simulink library "CTRL_SPECCTRL_COND"  (R2024b)
settings: Solver=VariableStepAuto  StartTime=0.0  StopTime=10.0  RelTol=1e-3
settings Model: Creator=blatak  LastModifiedBy=blatak

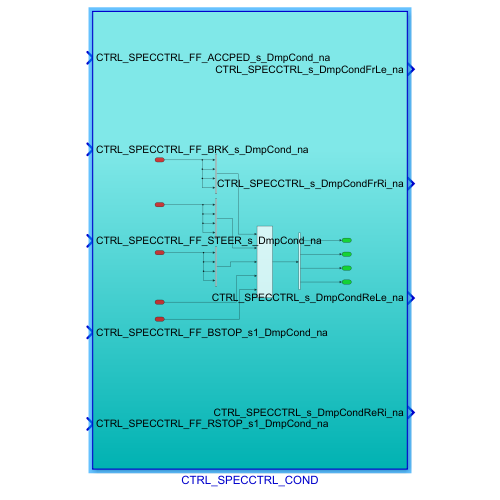
[thumbnail: Simulink's stored preview of the top-level diagram]
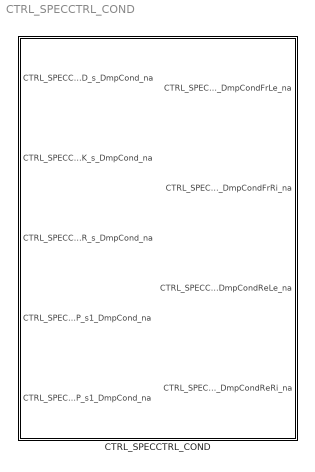
== system CTRL_SPECCTRL_COND ==
  CTRL_SPECCTRL_COND : Subsystem

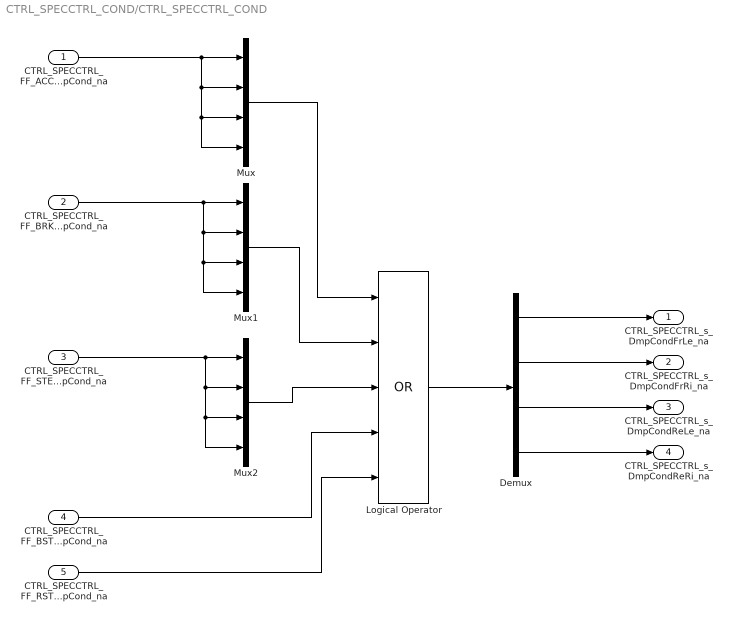
== system CTRL_SPECCTRL_COND/CTRL_SPECCTRL_COND ==
  CTRL_SPECCTRL_FF_ACCPED_s_DmpCond_na : Inport
  CTRL_SPECCTRL_FF_BRK_s_DmpCond_na : Inport  Port=2
  CTRL_SPECCTRL_FF_STEER_s_DmpCond_na : Inport  Port=3
  CTRL_SPECCTRL_FF_BSTOP_s1_DmpCond_na : Inport  Port=4
  CTRL_SPECCTRL_FF_RSTOP_s1_DmpCond_na : Inport  Port=5
  Demux : Demux
  Logical Operator : Logic  Operator=OR  Inputs=5  AllPortsSameDT=off  OutDataTypeStr=boolean
  Mux : Mux
  Mux1 : Mux
  Mux2 : Mux
  CTRL_SPECCTRL_s_DmpCondFrLe_na : Outport
  CTRL_SPECCTRL_s_DmpCondFrRi_na : Outport  Port=2
  CTRL_SPECCTRL_s_DmpCondReLe_na : Outport  Port=3
  CTRL_SPECCTRL_s_DmpCondReRi_na : Outport  Port=4
  wires:
  CTRL_SPECCTRL_FF_ACCPED_s_DmpCond_na/1 -> Mux/4, Mux/3, Mux/2, Mux/1
  CTRL_SPECCTRL_FF_BRK_s_DmpCond_na/1 -> Mux1/4, Mux1/3, Mux1/2, Mux1/1
  CTRL_SPECCTRL_FF_STEER_s_DmpCond_na/1 -> Mux2/4, Mux2/3, Mux2/2, Mux2/1
  Mux/1 -> Logical Operator/1
  Mux1/1 -> Logical Operator/2
  Mux2/1 -> Logical Operator/3
  CTRL_SPECCTRL_FF_BSTOP_s1_DmpCond_na/1 -> Logical Operator/4
  CTRL_SPECCTRL_FF_RSTOP_s1_DmpCond_na/1 -> Logical Operator/5
  Logical Operator/1 -> Demux/1
  Demux/1 -> CTRL_SPECCTRL_s_DmpCondFrLe_na/1
  Demux/2 -> CTRL_SPECCTRL_s_DmpCondFrRi_na/1
  Demux/3 -> CTRL_SPECCTRL_s_DmpCondReLe_na/1
  Demux/4 -> CTRL_SPECCTRL_s_DmpCondReRi_na/1
